simulink model "modulador_completo"  (R2020a)
settings: Solver=VariableStepAuto  StartTime=0.0  StopTime=10.0  RelTol=1e-3
model workspace: external: MATLAB File D:\Ferran\Facultad\UNCuyo\Meca\Automática y Máquinas Eléctricas\Proyecto final\matlab\parametros_y_especs\parametros_y_especif.m (data not in the file)
undefined symbols (not defined in the file): beq, lambda_m, Ld, Lq, Pp, R0, Rq, Rs
settings Model: Creator=Ferran  LastModifiedBy=Ferran

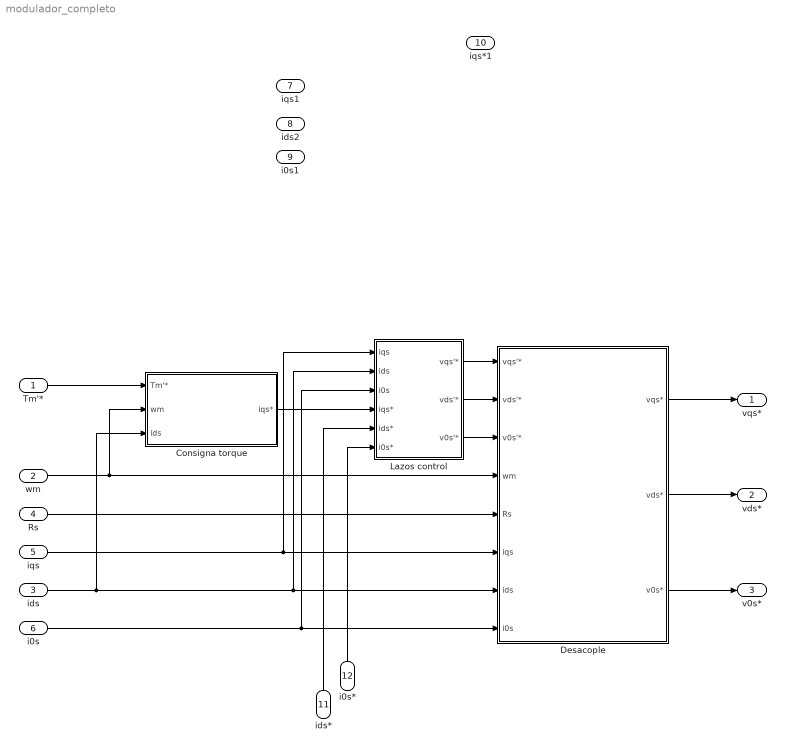
== system modulador_completo ==
  Tm'* : Inport
  wm : Inport  Port=2
  ids : Inport  Port=3
  Rs : Inport  Port=4
  iqs : Inport  Port=5
  i0s : Inport  Port=6
  iqs1 : Inport  Port=7
  ids2 : Inport  Port=8
  i0s1 : Inport  Port=9
  iqs*1 : Inport  Port=10
  ids* : Inport  Port=11
  i0s* : Inport  Port=12
  Consigna torque : Subsystem
  Desacople : Subsystem
  Lazos control : Subsystem
  vqs* : Outport
  vds* : Outport  Port=2
  v0s* : Outport  Port=3
  wires:
  Consigna torque/1(iqs*) -> Lazos control/4(iqs*)
  Lazos control/1(vqs'*) -> Desacople/1(vqs'*)
  Lazos control/2(vds'*) -> Desacople/2(vds'*)
  Lazos control/3(v0s'*) -> Desacople/3(v0s'*)
  Desacople/2(vds*) -> vds*/1
  Desacople/1(vqs*) -> vqs*/1
  Desacople/3(v0s*) -> v0s*/1
  wm/1 -> Consigna torque/2(wm), Desacople/4(wm)
  ids/1 -> Consigna torque/3(ids), Desacople/7(ids), Lazos control/2(ids)
  iqs/1 -> Desacople/6(iqs), Lazos control/1(iqs)
  i0s/1 -> Desacople/8(i0s), Lazos control/3(i0s)
  Rs/1 -> Desacople/5(Rs)
  Tm'*/1 -> Consigna torque/1(Tm'*)
  ids*/1 -> Lazos control/5(ids*)
  i0s*/1 -> Lazos control/6(i0s*)

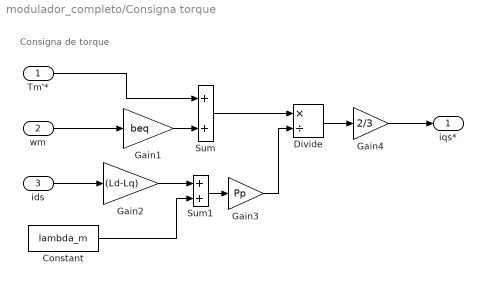
== system modulador_completo/Consigna torque ==
  note: Consigna de torque
  Tm'* : Inport
  wm : Inport  Port=2
  ids : Inport  Port=3
  Constant : Constant  Value=lambda_m
  Divide : Product  Inputs=*/
  Gain1 : Gain  Gain=beq
  Gain2 : Gain  Gain=(Ld-Lq)
  Gain3 : Gain  Gain=Pp
  Gain4 : Gain  Gain=2/3
  Sum : Sum
  Sum1 : Sum
  iqs* : Outport
  wires:
  Constant/1 -> Sum1/2
  Gain2/1 -> Sum1/1
  Tm'*/1 -> Sum/1
  Gain4/1 -> iqs*/1
  Divide/1 -> Gain4/1
  Sum1/1 -> Gain3/1
  Gain3/1 -> Divide/2
  Gain1/1 -> Sum/2
  Sum/1 -> Divide/1
  wm/1 -> Gain1/1
  ids/1 -> Gain2/1

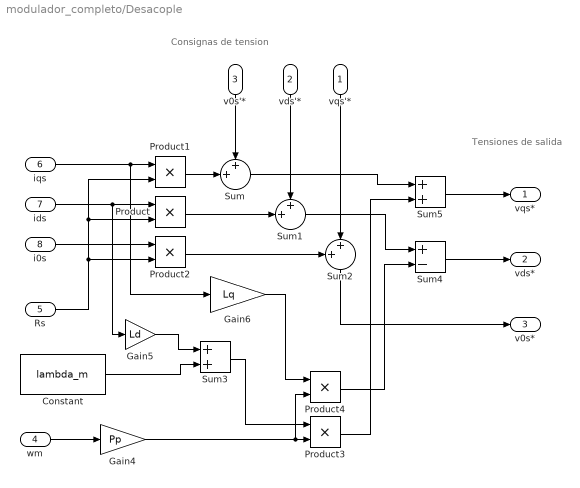
== system modulador_completo/Desacople ==
  note: Tensiones
      | de salida
  note: Consignas de tension
  vqs'* : Inport
  vds'* : Inport  Port=2
  v0s'* : Inport  Port=3
  wm : Inport  Port=4
  Rs : Inport  Port=5
  iqs : Inport  Port=6
  ids : Inport  Port=7
  i0s : Inport  Port=8
  Constant : Constant  Value=lambda_m
  Gain4 : Gain  Gain=Pp
  Gain5 : Gain  Gain=Ld
  Gain6 : Gain  Gain=Lq
  Product{,1..4} (5 alike) : Product
  Sum : Sum  Inputs=++|
  Sum1 : Sum  Inputs=++|
  Sum2 : Sum  Inputs=++|
  Sum3 : Sum
  Sum4 : Sum  Inputs=+-
  Sum5 : Sum
  vqs* : Outport
  vds* : Outport  Port=2
  v0s* : Outport  Port=3
  wires:
  vqs'*/1 -> Sum2/2
  Sum/1 -> Sum5/1
  Sum5/1 -> vqs*/1
  iqs/1 -> Product1/1, Gain6/1
  Product2/1 -> Sum2/1
  ids/1 -> Product/1, Gain5/1
  Gain4/1 -> Product4/2, Product3/2
  Product3/1 -> Sum5/2
  Rs/1 -> Product2/2, Product/2, Product1/2
  Product1/1 -> Sum/2
  Sum2/1 -> v0s*/1
  Sum4/1 -> vds*/1
  Constant/1 -> Sum3/2
  Gain5/1 -> Sum3/1
  Sum1/1 -> Sum4/1
  v0s'*/1 -> Sum/1
  i0s/1 -> Product2/1
  vds'*/1 -> Sum1/1
  Product4/1 -> Sum4/2
  Sum3/1 -> Product3/1
  wm/1 -> Gain4/1
  Product/1 -> Sum1/2
  Gain6/1 -> Product4/1

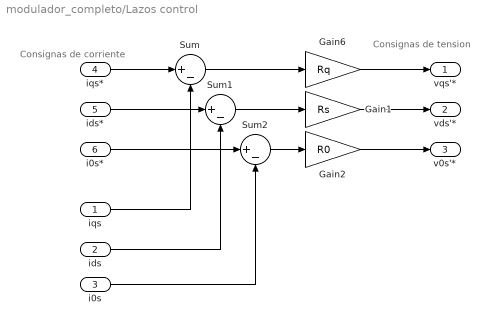
== system modulador_completo/Lazos control ==
  note: Consignas de tension
  note: Consignas
      | de
      | corriente
  iqs : Inport
  ids : Inport  Port=2
  i0s : Inport  Port=3
  iqs* : Inport  Port=4
  ids* : Inport  Port=5
  i0s* : Inport  Port=6
  Gain1 : Gain  Gain=Rs
  Gain2 : Gain  Gain=R0
  Gain6 : Gain  Gain=Rq
  Sum : Sum  Inputs=|+-
  Sum1 : Sum  Inputs=|+-
  Sum2 : Sum  Inputs=|+-
  vqs'* : Outport
  vds'* : Outport  Port=2
  v0s'* : Outport  Port=3
  wires:
  i0s*/1 -> Sum2/1
  i0s/1 -> Sum2/2
  Sum1/1 -> Gain1/1
  Gain6/1 -> vqs'*/1
  Sum/1 -> Gain6/1
  Sum2/1 -> Gain2/1
  Gain1/1 -> vds'*/1
  iqs*/1 -> Sum/1
  ids/1 -> Sum1/2
  iqs/1 -> Sum/2
  Gain2/1 -> v0s'*/1
  ids*/1 -> Sum1/1
